simulink model "NMPC_RAS"  (R2024a)
settings: Solver=ode4  StartTime=0.0  StopTime=10  FixedStep=Ts  RelTol=1e-3
values from neighbouring files (symbols this model uses):
  bs = 7.5    [initparams.m]
  bus = 5    [initparams.m]
  delta_Fc_max = 1000*Ts    (= 10)    [initparams.m]
  delta_Fc_min = -1000*Ts    (= -10)    [initparams.m]
  E = 1    [nmpc.m]    (also in nulmpc.m = 5)
  Fc_max = 15    [initparams.m]
  Fc_min = -15    [initparams.m]
  HcMB = 1    [nmpc.m]
  ks = 900    [initparams.m]
  kus = kt    (= 2500)    [initparams.m]
  ms = 2.45    [initparams.m]
  mus = mu    (= 1)    [initparams.m]
  n_max = 0.05    [initparams.m]
  n_min = -0.05    [initparams.m]
  Q_n = 10000    [nmpc.m]    (also in nulmpc.m = 1000)
  Q_ndot = 100    [nmpc.m]    (also in nulmpc.m = 5)
  R = 10    [nmpc.m]    (also in nulmpc.m)
  Ts = 0.01    [initparams.m]
  z1_dot_init = 0    [initparams.m]
  z1_init = 0.005    [initparams.m]
  z2_dot_init = 0    [initparams.m]
  z2_init = 0    [initparams.m]
libraries: simulink x1, mpclib x1
settings Model: Creator=aidan  LastModifiedBy=aidan
settings DebuggingCC: UnderSpecifiedDimensionMsg=warning

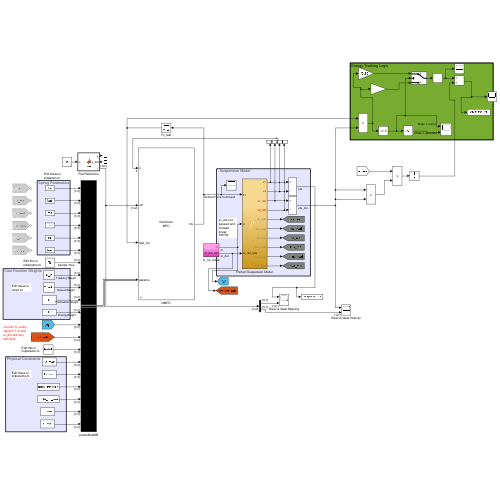
[thumbnail: Simulink's stored preview of the top-level diagram]
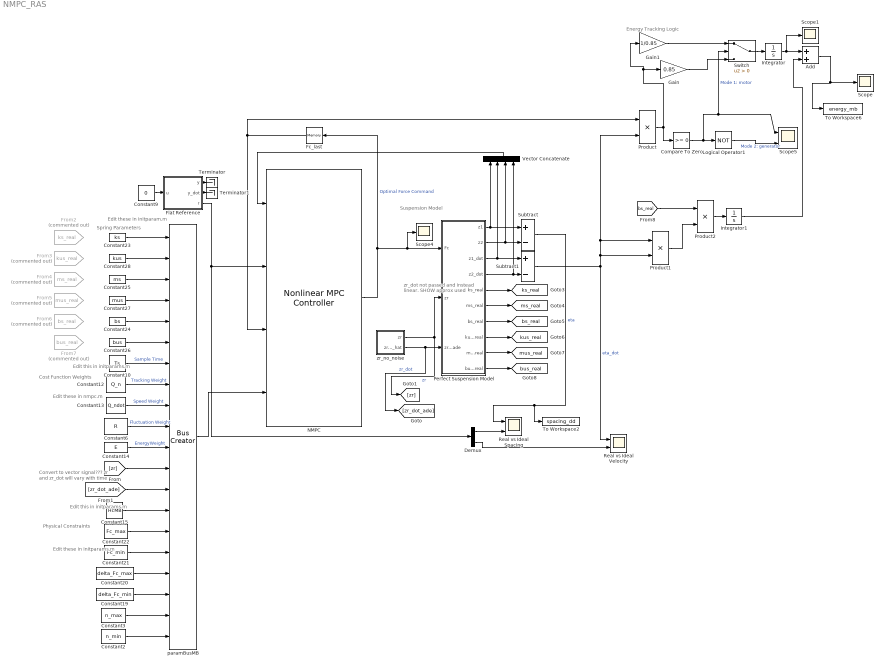
== system NMPC_RAS ==
  note: Convert to vector signal??? zr and zr_dot will vary with time
  note: zr_dot not passed and instead linear. SHOW approx used
  note: Edit these in initparam.m
  note: Physical Constraints
  note: Suspension Model
  note: Spring Parameters
  note: Cost Function Weights
  note: Energy Tracking Logic
  note: Edit these in nmpc.m
  note: Edit these in initparams.m
  note: Edit this in initparams.m
  note: Edit this in initparams.m
  Add : Sum
  Compare To Zero : simulink/Logic and Bit Operations/Compare To Zero  relop=>=  OutDataTypeStr=boolean
  Constant10 : Constant  Value=Ts
  Constant12 : Constant  Value=Q_n
  Constant13 : Constant  Value=Q_ndot
  Constant14 : Constant  Value=E
  Constant15 : Constant  Value=HcMB
  Constant19 : Constant  Value=delta_Fc_min
  Constant2 : Constant  Value=n_min
  Constant20 : Constant  Value=delta_Fc_max
  Constant21 : Constant  Value=Fc_min
  Constant22 : Constant  Value=Fc_max
  Constant23 : Constant  Value=ks
  Constant24 : Constant  Value=bs
  Constant25 : Constant  Value=ms
  Constant26 : Constant  Value=bus
  Constant27 : Constant  Value=mus
  Constant28 : Constant  Value=kus
  Constant3 : Constant  Value=n_max
  Constant6 : Constant  Value=R
  Constant9 : Constant  Value=0
  Demux : Demux  Outputs=2
  Fc_last : Memory  InheritSampleTime=on
  Flat Reference : MATLAB Function  TreatAsAtomicUnit=on
  From2 : From  Commented=on  GotoTag=ks_real  TagVisibility=global
  From3 : From  Commented=on  GotoTag=kus_real  TagVisibility=global
  From4 : From  Commented=on  GotoTag=ms_real  TagVisibility=global
  From5 : From  Commented=on  GotoTag=mus_real  TagVisibility=global
  From6 : From  Commented=on  GotoTag=bs_real  TagVisibility=global
  From7 : From  Commented=on  GotoTag=bus_real  TagVisibility=global
  Gain : Gain  Gain=0.85
  Gain1 : Gain  Gain=1/0.85
  Integrator : Integrator
  Integrator1 : Integrator
  Logical Operator1 : Logic  Operator=NOT  AllPortsSameDT=off  OutDataTypeStr=boolean
  NMPC : mpclib/Nonlinear MPC Controller  nlmpcobj=nmpcobj  UseObjectTs=on  UseMEX=off  md_enabled=off  mvtarget_enabled=off  param_enabled=on  cost_enabled=off  mvseq_enabled=off  stateseq_enabled=off  ovseq_enabled=off  slack_enabled=off  status_enabled=off  ov_min=off  ov_max=off  mv_min=off  mv_max=off  mvrate_min=off  mvrate_max=off  state_min=off  state_max=off  ov_weight=off  mv_weight=off  mvrate_weight=off  ecr_weight=off  nlp_initialize=off
  Perfect Suspension Model : Subsystem
  Product : Product
  Product1 : Product
  Product2 : Product
  Real vs Ideal Spacing : Scope  NumInputPorts=2
  Real vs Ideal Velocity : Scope  NumInputPorts=2
  Scope : Scope
  Scope1 : Scope
  Scope4 : Scope
  Scope5 : Scope  NumInputPorts=2
  Subtract : Sum  Inputs=+-
  Subtract1 : Sum  Inputs=+-
  Switch : Switch  Criteria=u2 > Threshold  SaturateOnIntegerOverflow=off  InputSameDT=off
  Terminator : Terminator
  Terminator1 : Terminator
  To Workspace2 : ToWorkspace  VariableName=spacing_dd  SaveFormat=Timeseries  SampleTime=-1
  To Workspace6 : ToWorkspace  VariableName=energy_mb  SaveFormat=Timeseries  SampleTime=-1
  Vector Concatenate : Concatenate  NumInputs=4
  paramBusMB : BusCreator  Inputs=20  OutDataTypeStr=Bus: paramBusMB  NonVirtualBus=on
      settings: InheritFromInputs=off
  zr_no_noise : Subsystem
  tag scope: bs_real=global, bus_real=global, ks_real=global, kus_real=global, ms_real=global, mus_real=global
  wires:
  Perfect Suspension Model/5(ks_real) -> [ks_real]
  Perfect Suspension Model/6(ms_real) -> [ms_real]
  Perfect Suspension Model/7(bs_real) -> [bs_real]
  Perfect Suspension Model/8(kus_real) -> [kus_real]
  Perfect Suspension Model/9(mus_real) -> [mus_real]
  Perfect Suspension Model/10(bus_real) -> [bus_real]
  Perfect Suspension Model/3(z1_dot) -> Subtract1/1, Vector Concatenate/2
  Perfect Suspension Model/4(z2_dot) -> Vector Concatenate/4, Subtract1/2
  Perfect Suspension Model/2(z2) -> Subtract/2, Vector Concatenate/3
  Subtract1/1 -> Product/2, Product1/1, Product1/2, Real vs Ideal Velocity/1  "eta_dot"
  Vector Concatenate/1 -> NMPC/1
  NMPC/1 -> Perfect Suspension Model/1(Fc), Scope4/1, Fc_last/1  "Optimal Force Command"
  Subtract/1 -> Real vs Ideal Spacing/1, To Workspace2/1  "eta"
  Constant9/1 -> Flat Reference/1(u)
  Flat Reference/2(y_dot) -> Terminator1/1
  Flat Reference/1(y) -> Terminator/1
  paramBusMB/1 -> NMPC/4
  Fc_last/1 -> NMPC/3, Product/1
  Flat Reference/3(r) -> Demux/1, NMPC/2
  Demux/1 -> Real vs Ideal Spacing/2
  Demux/2 -> Real vs Ideal Velocity/2
  Constant21/1 -> paramBusMB/16
  Constant22/1 -> paramBusMB/15
  Constant19/1 -> paramBusMB/18
  Constant20/1 -> paramBusMB/17
  Constant23/1 -> paramBusMB/1
  Constant26/1 -> paramBusMB/6
  Constant28/1 -> paramBusMB/2
  Constant25/1 -> paramBusMB/3
  Constant27/1 -> paramBusMB/4
  Constant24/1 -> paramBusMB/5
  Constant10/1 -> paramBusMB/7  "Sample Time"
  Constant12/1 -> paramBusMB/8  "Tracking Weight"
  Constant13/1 -> paramBusMB/9  "Speed Weight"
  Constant6/1 -> paramBusMB/10  "Fluctuation Weight"
  Constant14/1 -> paramBusMB/11  "EnergyWeight"
  Constant15/1 -> paramBusMB/14
  zr_no_noise/1(zr) -> Perfect Suspension Model/2(zr), [zr]  "zr"
  Perfect Suspension Model/1(z1) -> Subtract/1, Vector Concatenate/1
  Gain1/1 -> Switch/1
  Switch/1 -> Integrator/1
  Product/1 -> Compare To Zero/1, Gain/1, Gain1/1
  Compare To Zero/1 -> Scope5/1, Switch/2, Logical Operator1/1  "Mode 1: motor"
  Logical Operator1/1 -> Scope5/2  "Mode 2: generator"
  Gain/1 -> Switch/3
  [zr_dot_ade] -> paramBusMB/13
  [zr] -> paramBusMB/12
  zr_no_noise/2(zr_dot_hat) -> [zr_dot_ade], Perfect Suspension Model/3(zr_dot_ade)  "zr_dot"
  Constant2/1 -> paramBusMB/20
  Constant3/1 -> paramBusMB/19
  Product1/1 -> Product2/2
  [bs_real] -> Product2/1
  Product2/1 -> Integrator1/1
  Integrator1/1 -> Add/2
  Integrator/1 -> Scope1/1, Add/1
  Add/1 -> Scope/1, To Workspace6/1

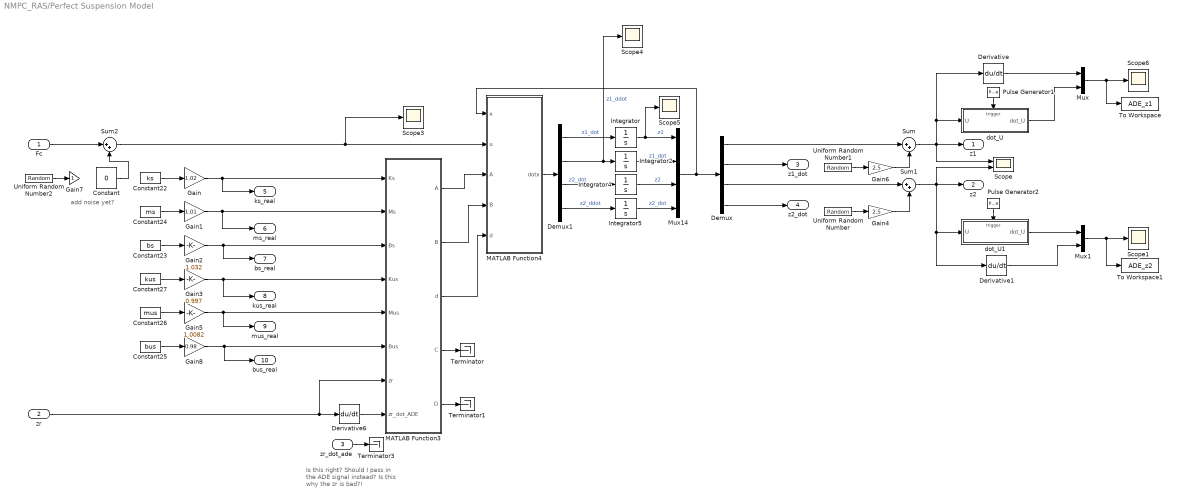
== system NMPC_RAS/Perfect Suspension Model ==
  note: Is this right? Should I pass in the ADE signal instead? Is this why the zr is bad?!
  note: add noise yet?
  Fc : Inport
  zr : Inport  Port=2
  zr_dot_ade : Inport  Port=3
  Constant : Constant  Value=0
  Constant22 : Constant  Value=ks
  Constant23 : Constant  Value=bs
  Constant24 : Constant  Value=ms
  Constant25 : Constant  Value=bus
  Constant26 : Constant  Value=mus
  Constant27 : Constant  Value=kus
  Demux : Demux
  Demux1 : Demux
  Derivative : Derivative
  Derivative1 : Derivative
  Derivative6 : Derivative
  Gain : Gain  Gain=1.02
  Gain1 : Gain  Gain=1.01
  Gain2 : Gain  Gain=1.032
  Gain3 : Gain  Gain=0.997
  Gain4 : Gain  Gain=2.5
  Gain5 : Gain  Gain=1.0082
  Gain6 : Gain  Gain=2.5
  Gain7 : Gain
  Gain8 : Gain  Gain=0.98
  Integrator : Integrator  InitialCondition=z1_init
  Integrator2 : Integrator  InitialCondition=z1_dot_init
  Integrator4 : Integrator  InitialCondition=z2_init
  Integrator5 : Integrator  InitialCondition=z2_dot_init
  MATLAB Function3 : MATLAB Function  TreatAsAtomicUnit=on
  MATLAB Function4 : MATLAB Function  TreatAsAtomicUnit=on
  Mux : Mux  Inputs=2
  Mux1 : Mux  Inputs=2
  Mux14 : Mux
  Pulse Generator1 : DiscretePulseGenerator  PulseType=Time based  Period=Ts*2  PulseWidth=50
  Pulse Generator2 : DiscretePulseGenerator  PulseType=Time based  Period=Ts*2  PulseWidth=50
  Scope : Scope  NumInputPorts=2
  Scope{1,3..6} (5 alike) : Scope
  Sum : Sum  Inputs=|++
  Sum1 : Sum  Inputs=|++
  Sum2 : Sum  Inputs=|++
  Terminator : Terminator
  Terminator1 : Terminator
  Terminator3 : Terminator
  To Workspace : ToWorkspace  VariableName=ADE_z1  SampleTime=-1
  To Workspace1 : ToWorkspace  VariableName=ADE_z2  SampleTime=-1
  Uniform Random Number : UniformRandomNumber  Minimum=-1e-6  Maximum=1e-6  Seed=244334  SampleTime=Ts
  Uniform Random Number1 : UniformRandomNumber  Minimum=-1e-6  Maximum=1e-6  Seed=7  SampleTime=Ts
  Uniform Random Number2 : UniformRandomNumber  Minimum=-5e-3  Maximum=5e-3  Seed=89757  SampleTime=Ts
  dot_U : Subsystem  TreatAsAtomicUnit=on
  dot_U1 : Subsystem  TreatAsAtomicUnit=on
  z1 : Outport
  z2 : Outport  Port=2
  z1_dot : Outport  Port=3
  z2_dot : Outport  Port=4
  ks_real : Outport  Port=5
  ms_real : Outport  Port=6
  bs_real : Outport  Port=7
  kus_real : Outport  Port=8
  mus_real : Outport  Port=9
  bus_real : Outport  Port=10
  wires:
  Constant23/1 -> Gain2/1
  MATLAB Function3/4(C) -> Terminator/1
  Demux1/1 -> Integrator/1  "z1_dot"
  zr/1 -> MATLAB Function3/7(zr), Derivative6/1
  Integrator5/1 -> Mux14/4  "z2_dot"
  Demux1/2 -> Scope4/1, Integrator2/1  "z1_ddot"
  Gain2/1 -> bs_real/1, MATLAB Function3/3(Bs)
  Constant27/1 -> Gain3/1
  Gain3/1 -> kus_real/1, MATLAB Function3/4(Kus)
  Constant24/1 -> Gain1/1
  Constant25/1 -> Gain8/1
  Demux1/4 -> Integrator5/1  "z2_ddot"
  MATLAB Function4/1(dotx) -> Demux1/1
  Integrator4/1 -> Mux14/3  "z2"
  Integrator/1 -> Scope5/1, Mux14/1  "z1"
  Constant26/1 -> Gain5/1
  Gain8/1 -> bus_real/1, MATLAB Function3/6(Bus)
  MATLAB Function3/2(B) -> MATLAB Function4/4(B)
  Constant22/1 -> Gain/1
  Demux1/3 -> Integrator4/1  "z2_dot"
  Gain5/1 -> mus_real/1, MATLAB Function3/5(Mus)
  MATLAB Function3/5(D) -> Terminator1/1
  Integrator2/1 -> Mux14/2  "z1_dot"
  Gain1/1 -> ms_real/1, MATLAB Function3/2(Ms)
  Gain/1 -> ks_real/1, MATLAB Function3/1(Ks)
  MATLAB Function3/1(A) -> MATLAB Function4/3(A)
  Mux14/1 -> Demux/1, MATLAB Function4/1(x)
  MATLAB Function3/3(d) -> MATLAB Function4/5(d)
  Demux/2 -> z1_dot/1
  Demux/4 -> z2_dot/1
  Gain4/1 -> Sum1/2
  Uniform Random Number/1 -> Gain4/1
  Sum/1 -> Scope/1, Derivative/1, dot_U/1(U), z1/1
  Demux/1 -> Sum/1
  Demux/3 -> Sum1/1
  Uniform Random Number1/1 -> Gain6/1
  Gain6/1 -> Sum/2
  dot_U/1(dot_U) -> Mux/2
  Pulse Generator1/1 -> dot_U/Trigger
  Derivative/1 -> Mux/1
  Pulse Generator2/1 -> dot_U1/Trigger
  Sum1/1 -> Scope/2, Derivative1/1, dot_U1/1(U), z2/1
  dot_U1/1(dot_U) -> Mux1/1
  Derivative1/1 -> Mux1/2
  Sum2/1 -> Scope3/1, MATLAB Function4/2(u)
  Fc/1 -> Sum2/1
  Uniform Random Number2/1 -> Gain7/1
  Mux/1 -> To Workspace/1, Scope6/1
  Mux1/1 -> Scope1/1, To Workspace1/1
  Constant/1 -> Sum2/2
  zr_dot_ade/1 -> Terminator3/1
  Derivative6/1 -> MATLAB Function3/8(zr_dot_ADE)

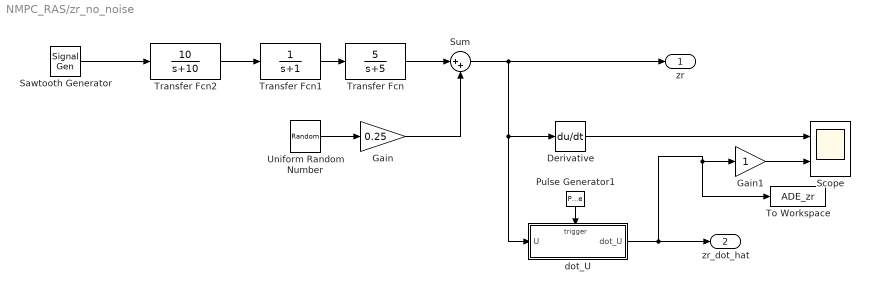
== system NMPC_RAS/zr_no_noise ==
  Derivative : Derivative
  Gain : Gain  Gain=0.25
  Gain1 : Gain
  Pulse Generator1 : DiscretePulseGenerator  PulseType=Time based  Period=Ts*2  PulseWidth=50
  Sawtooth Generator : SignalGenerator  WaveForm=sawtooth  Amplitude=3.5e-2
  Scope : Scope  NumInputPorts=2
  Sum : Sum  Inputs=|++
  To Workspace : ToWorkspace  VariableName=ADE_zr  SampleTime=-1
  Transfer Fcn : TransferFcn  Numerator=[5]  Denominator=[1 5]
  Transfer Fcn1 : TransferFcn  Denominator=[1 1]
  Transfer Fcn2 : TransferFcn  Numerator=[10]  Denominator=[1 10]
  Uniform Random Number : UniformRandomNumber  Minimum=-1e-6  Maximum=1e-6  Seed=122334  SampleTime=Ts
  dot_U : Subsystem  TreatAsAtomicUnit=on
  zr : Outport
  zr_dot_hat : Outport  Port=2
  wires:
  Transfer Fcn2/1 -> Transfer Fcn1/1
  Transfer Fcn/1 -> Sum/1
  Sawtooth Generator/1 -> Transfer Fcn2/1
  Transfer Fcn1/1 -> Transfer Fcn/1
  Uniform Random Number/1 -> Gain/1
  Gain/1 -> Sum/2
  Sum/1 -> dot_U/1(U), Derivative/1, zr/1
  Pulse Generator1/1 -> dot_U/Trigger
  Derivative/1 -> Scope/1
  dot_U/1(dot_U) -> To Workspace/1, Gain1/1, zr_dot_hat/1
  Gain1/1 -> Scope/2

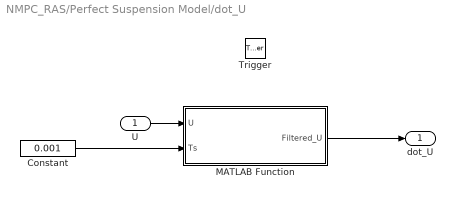
== system NMPC_RAS/Perfect Suspension Model/dot_U ==
  U : Inport
  Trigger : TriggerPort  TriggerType=either  VariantControl=Variant  ZeroCross=off  PortDimensions=1
  Constant : Constant  Value=0.001
  MATLAB Function : MATLAB Function  TreatAsAtomicUnit=on
  dot_U : Outport  VectorParamsAs1DForOutWhenUnconnected=off
  wires:
  Constant/1 -> MATLAB Function/2(Ts)
  MATLAB Function/1(Filtered_U) -> dot_U/1
  U/1 -> MATLAB Function/1(U)

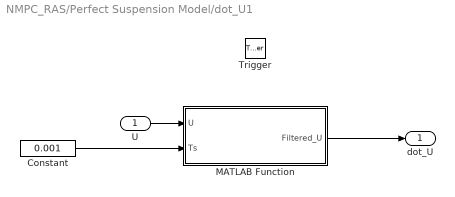
== system NMPC_RAS/Perfect Suspension Model/dot_U1 ==
  U : Inport
  Trigger : TriggerPort  TriggerType=either  VariantControl=Variant  ZeroCross=off  PortDimensions=1
  Constant : Constant  Value=0.001
  MATLAB Function : MATLAB Function  TreatAsAtomicUnit=on
  dot_U : Outport  VectorParamsAs1DForOutWhenUnconnected=off
  wires:
  U/1 -> MATLAB Function/1(U)
  MATLAB Function/1(Filtered_U) -> dot_U/1
  Constant/1 -> MATLAB Function/2(Ts)

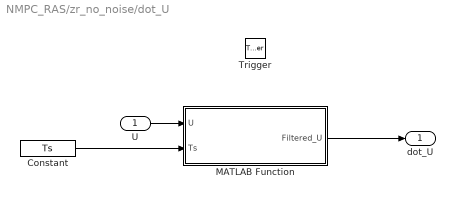
== system NMPC_RAS/zr_no_noise/dot_U ==
  U : Inport
  Trigger : TriggerPort  TriggerType=either  VariantControl=Variant  ZeroCross=off  PortDimensions=1
  Constant : Constant  Value=Ts
  MATLAB Function : MATLAB Function  TreatAsAtomicUnit=on
  dot_U : Outport  VectorParamsAs1DForOutWhenUnconnected=off
  wires:
  Constant/1 -> MATLAB Function/2(Ts)
  MATLAB Function/1(Filtered_U) -> dot_U/1
  U/1 -> MATLAB Function/1(U)

== matlab function NMPC_RAS/Perfect Suspension Model/MATLAB Function3 ==
  data: Ks input; A output; Ms input; Bs input; Kus input; Mus input; Bus input; zr input; zr_dot_ADE input; B output; d output; C output; D output
function [A, B, d, C, D] = Syst(Ks, Ms, Bs, Kus, Mus, Bus, zr, zr_dot_ADE)
    A = [    0,      1,             0,              0; 
        -Ks/Ms, -Bs/Ms,         Ks/Ms,          Bs/Ms; 
             0,      0,             0,              1; 
        Ks/Mus, Bs/Mus, -(Kus+Ks)/Mus, -(Bus+Bs)/Mus];
 
    
    B = [0; 1/Ms; 0; -1/Mus];
    
    
    d = [0;    0; 0;  Kus/Mus*zr + Bus/Mus*zr_dot_ADE];
   
    
    C = [    1,      0,    -1,     0;
        -Ks/Ms, -Bs/Ms, Ks/Ms, Bs/Ms];
    
    D = [0; 1/Ms];
    
    
end

== matlab function NMPC_RAS/zr_no_noise/dot_U/MATLAB Function ==
  data: U input; Filtered_U output; Ts input
function Filtered_U = buffer(U,Ts)
    N = 12;
    %Ts = 0.001;
    persistent y;
    if isempty(y)
        y=zeros(N+1,1);
    end

    y = [U;y(1:end-1)];
    T = Ts*N;
    P = zeros(1,N+1);
    P_alpha = P;
    for k = 1:N+1
        tao_k = (k-1)*Ts;
        P(k) = T-2*tao_k;
        if((k==1)||(k==N+1))
            P_alpha(k) = P(k)*Ts/2;
        else
            P_alpha(k) = P(k)*Ts;
        end
    end
    
    Filtered_U = P_alpha*y*6/(T^3);

end

== matlab function NMPC_RAS/Perfect Suspension Model/dot_U/MATLAB Function ==
  data: U input; Filtered_U output; Ts input
function Filtered_U = buffer(U,Ts)
    N = 10;
    %Ts = 0.001;
    persistent y;
    if isempty(y)
        y=zeros(N+1,1);
    end

    y = [U;y(1:end-1)];
    T = Ts*N;
    P = zeros(1,N+1);
    P_alpha = P;
    for k = 1:N+1
        tao_k = (k-1)*Ts;
        P(k) = T-2*tao_k;
        if((k==1)||(k==N+1))
            P_alpha(k) = P(k)*Ts/2;
        else
            P_alpha(k) = P(k)*Ts;
        end
    end
    
    Filtered_U = P_alpha*y*6/(T^3);

end

== matlab function NMPC_RAS/Perfect Suspension Model/dot_U1/MATLAB Function ==
  data: U input; Filtered_U output; Ts input
function Filtered_U = buffer(U,Ts)
    N = 10;
    %Ts = 0.001;
    persistent y;
    if isempty(y)
        y=zeros(N+1,1);
    end

    y = [U;y(1:end-1)];
    T = Ts*N;
    P = zeros(1,N+1);
    P_alpha = P;
    for k = 1:N+1
        tao_k = (k-1)*Ts;
        P(k) = T-2*tao_k;
        if((k==1)||(k==N+1))
            P_alpha(k) = P(k)*Ts/2;
        else
            P_alpha(k) = P(k)*Ts;
        end
    end
    
    Filtered_U = P_alpha*y*6/(T^3);

end

== matlab function NMPC_RAS/Flat Reference ==
  data: u input; y output; y_dot output; r output
function [y, y_dot, r]= fcn(u)

y = u;
y_dot = 0;
% r = [y;y_dot];
r = [y,y_dot];

== matlab function NMPC_RAS/Perfect Suspension Model/MATLAB Function4 ==
  data: x input; dotx output; u input; A input; B input; d input
function dotx  = Susp_System(x, u, A, B, d)
    
    dotx = A*x + B*u + d;
    %y = C*x + D*u;
end
